simulink model "liner_two_wheel_model"  (R2018a)
settings: Solver=ode4  StartTime=0.0  StopTime=100  FixedStep=0.001  RelTol=1e-3
values from neighbouring files (symbols this model uses):
  CORNERING_POWER_OF_FRONT_TIRE = 200/(pi/180)    (= 11459.1559026)    [PARAMETERS.m]
  CORNERING_POWER_OF_REAR_TIRE = 200/(pi/180)    (= 11459.1559026)    [PARAMETERS.m]
  FRONT_SIDE_WHEELBASE = 0.8    [PARAMETERS.m]
  GEAR_RATIO = 14    [PARAMETERS.m]
  GRAVITATIONAL_ACCELERATION = 9.8    [PARAMETERS.m]
  HEIGHT_OF_GRAVITIONAL_CENTER = 0.3    [PARAMETERS.m]
  INITIAL_VELOCITY = TARGET_VELOCITY    (= 18)    [PARAMETERS.m]
  MAX_MOTOR_TORQUE = 21    [PARAMETERS.m]
  MAX_STEERING_ANGLE = 20/180*pi    (= 0.349065850399)    [PARAMETERS.m]
  REAR_SIDE_WHEELBASE = 0.7    [PARAMETERS.m]
  TIRE_RADIUS = 0.2286    [PARAMETERS.m]
  VEHICLE_MASS = 300    [PARAMETERS.m]
  VEHICLE_YAW_INERTIA = 120    [PARAMETERS.m]
  WHEELBASE = 1.5    [PARAMETERS.m]
libraries: simulink x1
settings Model: Creator=kntys  LastModifiedBy=kntys

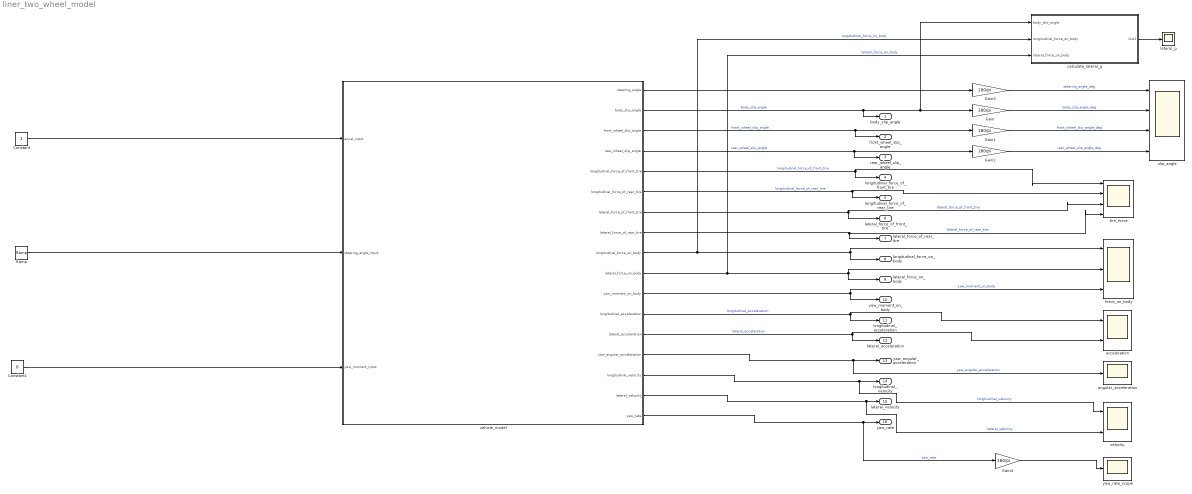
== system liner_two_wheel_model ==
  Constant : Constant
  Constant1 : Constant  Value=0
  Gain{,1..4} (5 alike) : Gain  Gain=180/pi
  Ramp : simulink/Sources/Ramp  slope=0.01  start=0  InitialOutput=0
  acceleration : Scope  NumInputPorts=2
  angular_acceleration : Scope
  calculate_lateral_g : Subsystem
  force_on_body : Scope  NumInputPorts=3
  lateral_g : Scope
  slip_angle : Scope  NumInputPorts=4
  tire_force : Scope  NumInputPorts=4
  vehicle_model : Subsystem
  velocity : Scope  NumInputPorts=2
  yaw_rate_scope : Scope
  body_slip_angle : Outport
  front_wheel_slip_angle : Outport  Port=2
  rear_wheel_slip_angle : Outport  Port=3
  longitudinal_force_of_front_tire : Outport  Port=4
  longitudinal_force_of_rear_tire : Outport  Port=5
  lateral_force_of_front_tire : Outport  Port=6
  lateral_force_of_rear_tire : Outport  Port=7
  longitudinal_force_on_body : Outport  Port=8
  lateral_force_on_body : Outport  Port=9
  yaw_moment_on_body : Outport  Port=10
  longitudinal_acceleration : Outport  Port=11
  lateral_acceleration : Outport  Port=12
  yaw_angular_acceleration : Outport  Port=13
  longitudinal_velocity : Outport  Port=14
  lateral_velocity : Outport  Port=15
  yaw_rate : Outport  Port=16
  wires:
  Ramp/1 -> vehicle_model/2(steering_angle_input)
  vehicle_model/16(lateral_velocity) -> velocity/2, lateral_velocity/1  "lateral_velocity"
  vehicle_model/15(longitudinal_velocity) -> velocity/1, longitudinal_velocity/1  "longitudinal_velocity"
  vehicle_model/17(yaw_rate) -> Gain4/1, yaw_rate/1  "yaw_rate"
  vehicle_model/2(body_slip_angle) -> body_slip_angle/1, calculate_lateral_g/1(body_slip_angle), Gain/1  "body_slip_angle"
  vehicle_model/3(front_wheel_slip_angle) -> front_wheel_slip_angle/1, Gain1/1  "front_wheel_slip_angle"
  vehicle_model/4(rear_wheel_slip_angle) -> rear_wheel_slip_angle/1, Gain2/1  "rear_wheel_slip_angle"
  vehicle_model/5(longitudinal_force_of_front_tire) -> longitudinal_force_of_front_tire/1, tire_force/1  "longitudinal_force_of_front_tire"
  vehicle_model/6(longitudinal_force_of_rear_tire) -> longitudinal_force_of_rear_tire/1, tire_force/2  "longitudinal_force_of_rear_tire"
  vehicle_model/7(lateral_force_of_front_tire) -> lateral_force_of_front_tire/1, tire_force/3  "lateral_force_of_front_tire"
  vehicle_model/8(lateral_force_of_rear_tire) -> lateral_force_of_rear_tire/1, tire_force/4  "lateral_force_of_rear_tire"
  vehicle_model/9(longitudinal_force_on_body) -> calculate_lateral_g/2(longitudinal_force_on_body), longitudinal_force_on_body/1, force_on_body/1  "longitudinal_force_on_body"
  vehicle_model/10(lateral_force_on_body) -> calculate_lateral_g/3(lateral_force_on_body), lateral_force_on_body/1, force_on_body/2  "lateral_force_on_body"
  vehicle_model/11(yaw_moment_on_body) -> yaw_moment_on_body/1, force_on_body/3  "yaw_moment_on_body"
  vehicle_model/12(longitudinal_acceleration) -> longitudinal_acceleration/1, acceleration/1  "longitudinal_acceleration"
  vehicle_model/13(lateral_acceleration) -> lateral_acceleration/1, acceleration/2  "lateral_acceleration"
  vehicle_model/14(yaw_angular_acceleration) -> angular_acceleration/1, yaw_angular_acceleration/1  "yaw_angular_acceleration"
  Constant1/1 -> vehicle_model/3(yaw_moment_input)
  Constant/1 -> vehicle_model/1(accel_input)
  Gain/1 -> slip_angle/2  "body_slip_angle_deg"
  Gain1/1 -> slip_angle/3  "front_wheel_slip_angle_deg"
  Gain2/1 -> slip_angle/4  "rear_wheel_slip_angle_deg"
  vehicle_model/1(steering_angle) -> Gain3/1
  Gain3/1 -> slip_angle/1  "steering_angle_deg"
  Gain4/1 -> yaw_rate_scope/1
  calculate_lateral_g/1(Out1) -> lateral_g/1

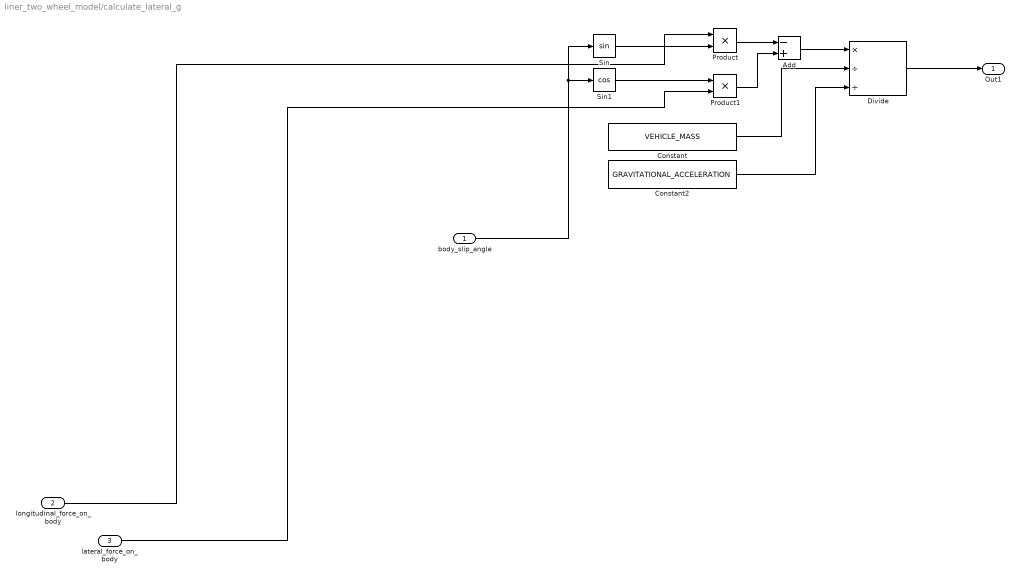
== system liner_two_wheel_model/calculate_lateral_g ==
  body_slip_angle : Inport
  longitudinal_force_on_body : Inport  Port=2
  lateral_force_on_body : Inport  Port=3
  Add : Sum  Inputs=-+
  Constant : Constant  Value=VEHICLE_MASS
  Constant2 : Constant  Value=GRAVITATIONAL_ACCELERATION
  Divide : Product  Inputs=*//
  Product : Product
  Product1 : Product
  Sin : Trigonometry
  Sin1 : Trigonometry  Operator=cos
  Out1 : Outport
  wires:
  body_slip_angle/1 -> Sin/1, Sin1/1
  Product/1 -> Add/1
  lateral_force_on_body/1 -> Product1/2
  Divide/1 -> Out1/1
  Add/1 -> Divide/1
  Constant2/1 -> Divide/3
  Sin1/1 -> Product1/1
  Constant/1 -> Divide/2
  Product1/1 -> Add/2
  Sin/1 -> Product/2
  longitudinal_force_on_body/1 -> Product/1

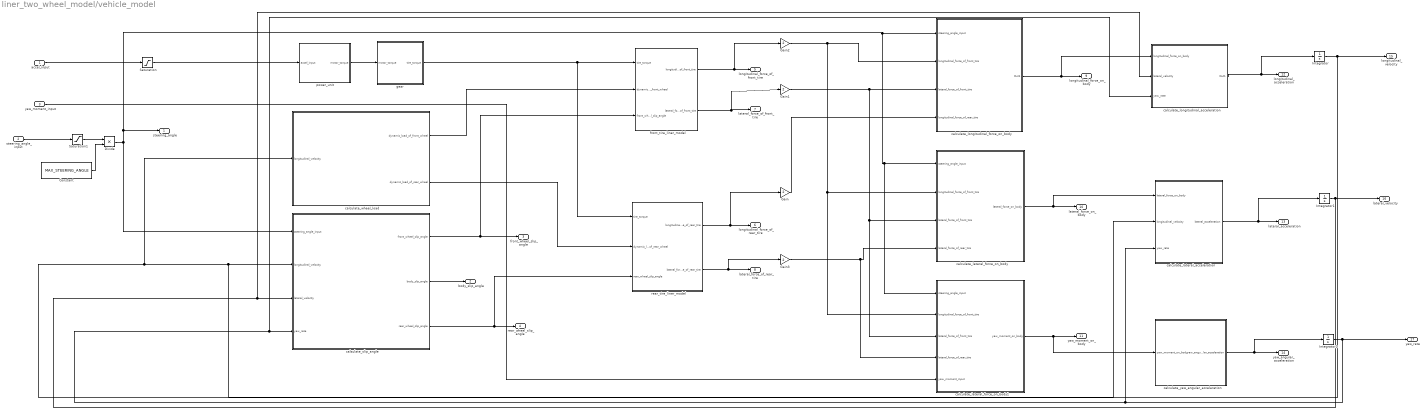
== system liner_two_wheel_model/vehicle_model ==
  accel_input : Inport
  steering_angle_input : Inport  Port=2
  yaw_moment_input : Inport  Port=3
  Constant : Constant  Value=MAX_STEERING_ANGLE
  Divide : Product  Inputs=**
  Gain{,1..3} (4 alike) : Gain  Gain=2
  Integrator : Integrator  InitialCondition=INITIAL_VELOCITY
  Integrator1 : Integrator
  Integrator2 : Integrator
  Saturation : Saturate  UpperLimit=1  LowerLimit=-1
  Saturation1 : Saturate  UpperLimit=1  LowerLimit=-1
  calculate_lateral_acceleration : Subsystem
  calculate_lateral_force_on_body : Subsystem
  calculate_lateral_force_on_body1 : Subsystem
  calculate_longitudinal_acceleration : Subsystem
  calculate_longitudinal_force_on_body : Subsystem
  calculate_wheel_load : Subsystem
  calculate_yaw_angular_accelaration : Subsystem
  calsulate_slip_angle : Subsystem
  front_tire_liner_model : Subsystem
  gear : Subsystem
  power_unit : Subsystem
  rear_tire_liner_model : Subsystem
  steering_angle : Outport
  body_slip_angle : Outport  Port=2
  front_wheel_slip_angle : Outport  Port=3
  rear_wheel_slip_angle : Outport  Port=4
  longitudinal_force_of_front_tire : Outport  Port=5
  longitudinal_force_of_rear_tire : Outport  Port=6
  lateral_force_of_front_tire : Outport  Port=7
  lateral_force_of_rear_tire : Outport  Port=8
  longitudinal_force_on_body : Outport  Port=9
  lateral_force_on_body : Outport  Port=10
  yaw_moment_on_body : Outport  Port=11
  longitudinal_acceleration : Outport  Port=12
  lateral_acceleration : Outport  Port=13
  yaw_angular_acceleration : Outport  Port=14
  longitudinal_velocity : Outport  Port=15
  lateral_velocity : Outport  Port=16
  yaw_rate : Outport  Port=17
  wires:
  accel_input/1 -> Saturation/1
  calculate_yaw_angular_accelaration/1(yaw_angular_acceleration) -> yaw_angular_acceleration/1, Integrator2/1
  Saturation/1 -> power_unit/1(accel_input)
  gear/1(tire_torque) -> rear_tire_liner_model/1(tire_torque), front_tire_liner_model/1(tire_torque)
  Gain/1 -> calculate_longitudinal_force_on_body/4(longitudinal_force_of_rear_tire)
  front_tire_liner_model/2(lateral_force_of_front_tire) -> lateral_force_of_front_tire/1, Gain1/1
  Gain2/1 -> calculate_lateral_force_on_body1/2(longitudinal_force_of_front_tire), calculate_lateral_force_on_body/2(longitudinal_force_of_front_tire), calculate_longitudinal_force_on_body/2(longitudinal_force_of_front_tire)
  calsulate_slip_angle/3(rear_wheel_slip_angle) -> rear_wheel_slip_angle/1, rear_tire_liner_model/3(rear_wheel_slip_angle)
  calculate_lateral_acceleration/1(lateral_acceleration) -> lateral_acceleration/1, Integrator1/1
  front_tire_liner_model/1(longitudinal_force_of_front_tire) -> longitudinal_force_of_front_tire/1, Gain2/1
  calsulate_slip_angle/1(front_wheel_slip_angle) -> front_wheel_slip_angle/1, front_tire_liner_model/3(front_wheel_slip_angle)
  Divide/1 -> calsulate_slip_angle/1(steering_angle_input), steering_angle/1, calculate_lateral_force_on_body1/1(steering_angle_input), calculate_lateral_force_on_body/1(steering_angle_input), calculate_longitudinal_force_on_body/1(steering_angle_input)
  calculate_longitudinal_acceleration/1(Out1) -> longitudinal_acceleration/1, Integrator/1
  calculate_wheel_load/2(dynamic_load_of_rear_wheel) -> rear_tire_liner_model/2(dynamic_load_of_rear_wheel)
  Integrator2/1 -> calculate_longitudinal_acceleration/3(yaw_rate), calsulate_slip_angle/4(yaw_rate), calculate_lateral_acceleration/3(yaw_rate), yaw_rate/1
  calculate_wheel_load/1(dynamic_load_of_front_wheel) -> front_tire_liner_model/2(dynamic_load_of_front_wheel)
  calsulate_slip_angle/2(body_slip_angle) -> body_slip_angle/1
  rear_tire_liner_model/2(lateral_force_of_rear_tire) -> lateral_force_of_rear_tire/1, Gain3/1
  Gain3/1 -> calculate_lateral_force_on_body1/4(lateral_force_of_rear_tire), calculate_lateral_force_on_body/4(lateral_force_of_rear_tire)
  rear_tire_liner_model/1(longitudinal_force_of_rear_tire) -> longitudinal_force_of_rear_tire/1, Gain/1
  calculate_lateral_force_on_body1/1(yaw_moment_on_body) -> yaw_moment_on_body/1, calculate_yaw_angular_accelaration/1(yaw_moment_on_body)
  Gain1/1 -> calculate_lateral_force_on_body1/3(lateral_force_of_front_tire), calculate_lateral_force_on_body/3(lateral_force_of_front_tire), calculate_longitudinal_force_on_body/3(lateral_force_of_front_tire)
  Integrator/1 -> longitudinal_velocity/1, calculate_wheel_load/1(longitudinal_velocity), calculate_lateral_acceleration/2(longitudinal_velocity), calsulate_slip_angle/2(longitudinal_velocity)
  calculate_lateral_force_on_body/1(lateral_force_on_body) -> lateral_force_on_body/1, calculate_lateral_acceleration/1(lateral_force_on_body)
  Integrator1/1 -> lateral_velocity/1, calculate_longitudinal_acceleration/2(lateral_velocity), calsulate_slip_angle/3(lateral_velocity)
  calculate_longitudinal_force_on_body/1(Out1) -> longitudinal_force_on_body/1, calculate_longitudinal_acceleration/1(longitudinal_force_on_body)
  yaw_moment_input/1 -> calculate_lateral_force_on_body1/5(yaw_moment_input)
  power_unit/1(motor_torque) -> gear/1(motor_torque)
  steering_angle_input/1 -> Saturation1/1
  Constant/1 -> Divide/2
  Saturation1/1 -> Divide/1

== system liner_two_wheel_model/vehicle_model/calculate_lateral_acceleration ==
  lateral_force_on_body : Inport
  longitudinal_velocity : Inport  Port=2
  yaw_rate : Inport  Port=3
  Add1 : Sum  Inputs=+-
  Constant1 : Constant  Value=VEHICLE_MASS
  Divide : Product  Inputs=*/
  Divide3 : Product  Inputs=**
  lateral_acceleration : Outport
  wires:
  longitudinal_velocity/1 -> Divide3/1
  Divide/1 -> Add1/1
  lateral_force_on_body/1 -> Divide/1
  Constant1/1 -> Divide/2
  yaw_rate/1 -> Divide3/2
  Add1/1 -> lateral_acceleration/1
  Divide3/1 -> Add1/2

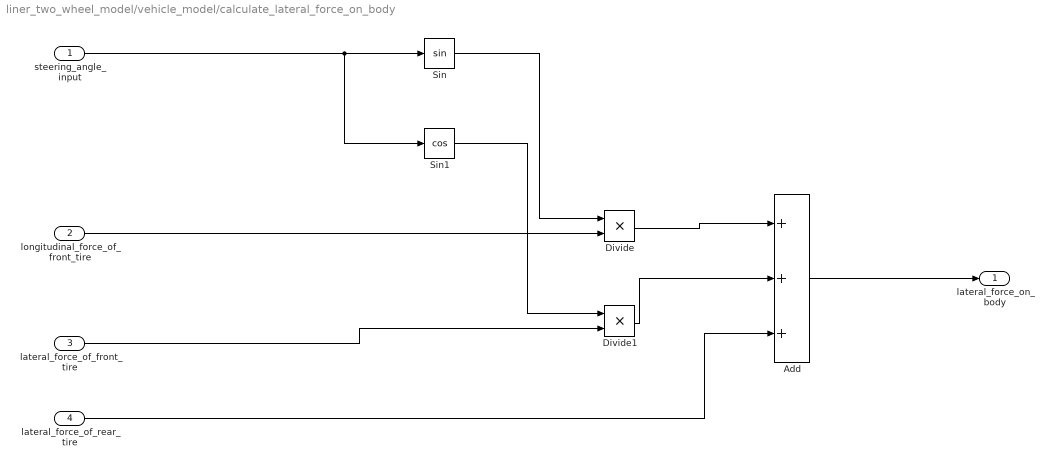
== system liner_two_wheel_model/vehicle_model/calculate_lateral_force_on_body ==
  steering_angle_input : Inport
  longitudinal_force_of_front_tire : Inport  Port=2
  lateral_force_of_front_tire : Inport  Port=3
  lateral_force_of_rear_tire : Inport  Port=4
  Add : Sum  Inputs=+++
  Divide : Product  Inputs=**
  Divide1 : Product  Inputs=**
  Sin : Trigonometry
  Sin1 : Trigonometry  Operator=cos
  lateral_force_on_body : Outport
  wires:
  longitudinal_force_of_front_tire/1 -> Divide/2
  steering_angle_input/1 -> Sin/1, Sin1/1
  Divide/1 -> Add/1
  Add/1 -> lateral_force_on_body/1
  Divide1/1 -> Add/2
  Sin1/1 -> Divide1/1
  Sin/1 -> Divide/1
  lateral_force_of_front_tire/1 -> Divide1/2
  lateral_force_of_rear_tire/1 -> Add/3

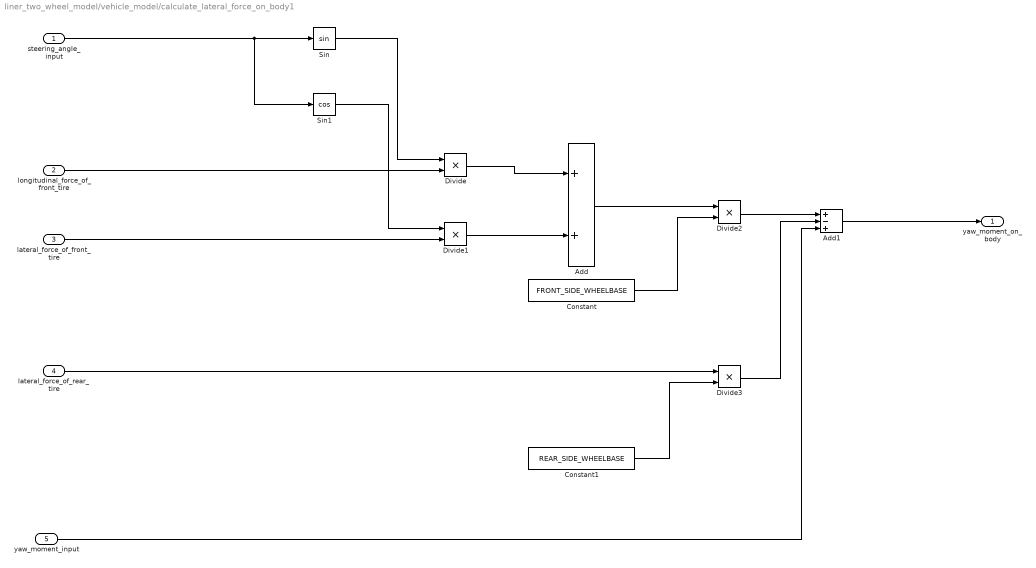
== system liner_two_wheel_model/vehicle_model/calculate_lateral_force_on_body1 ==
  steering_angle_input : Inport
  longitudinal_force_of_front_tire : Inport  Port=2
  lateral_force_of_front_tire : Inport  Port=3
  lateral_force_of_rear_tire : Inport  Port=4
  yaw_moment_input : Inport  Port=5
  Add : Sum
  Add1 : Sum  Inputs=+-+
  Constant : Constant  Value=FRONT_SIDE_WHEELBASE
  Constant1 : Constant  Value=REAR_SIDE_WHEELBASE
  Divide{,1..3} (4 alike) : Product  Inputs=**
  Sin : Trigonometry
  Sin1 : Trigonometry  Operator=cos
  yaw_moment_on_body : Outport
  wires:
  longitudinal_force_of_front_tire/1 -> Divide/2
  steering_angle_input/1 -> Sin/1, Sin1/1
  Divide/1 -> Add/1
  Add/1 -> Divide2/1
  Divide1/1 -> Add/2
  Sin1/1 -> Divide1/1
  Sin/1 -> Divide/1
  lateral_force_of_front_tire/1 -> Divide1/2
  lateral_force_of_rear_tire/1 -> Divide3/1
  Constant/1 -> Divide2/2
  Divide2/1 -> Add1/1
  Divide3/1 -> Add1/2
  Constant1/1 -> Divide3/2
  yaw_moment_input/1 -> Add1/3
  Add1/1 -> yaw_moment_on_body/1

== system liner_two_wheel_model/vehicle_model/calculate_longitudinal_acceleration ==
  longitudinal_force_on_body : Inport
  lateral_velocity : Inport  Port=2
  yaw_rate : Inport  Port=3
  Add : Sum
  Constant : Constant  Value=VEHICLE_MASS
  Divide1 : Product  Inputs=*/
  Divide2 : Product  Inputs=**
  Out1 : Outport
  wires:
  Divide1/1 -> Add/1
  longitudinal_force_on_body/1 -> Divide1/1
  lateral_velocity/1 -> Divide2/1
  Divide2/1 -> Add/2
  yaw_rate/1 -> Divide2/2
  Constant/1 -> Divide1/2
  Add/1 -> Out1/1

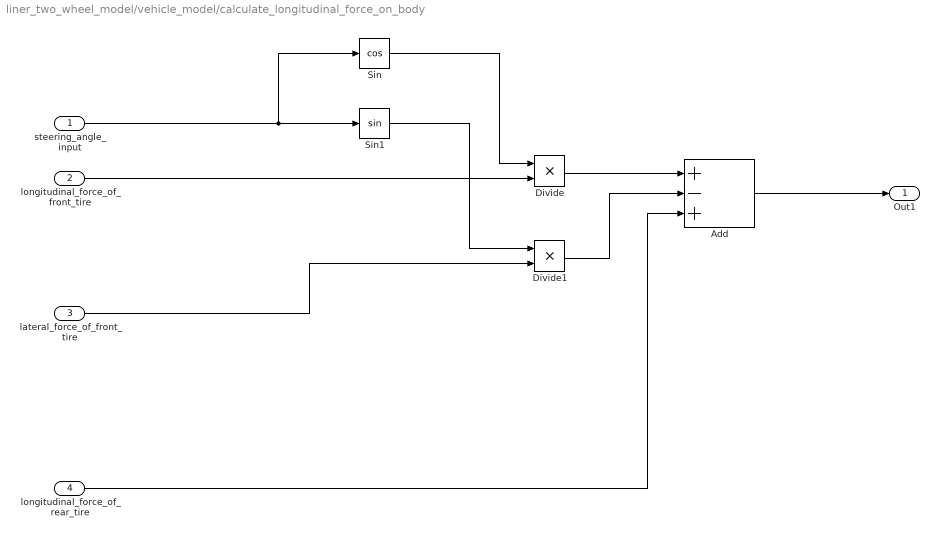
== system liner_two_wheel_model/vehicle_model/calculate_longitudinal_force_on_body ==
  steering_angle_input : Inport
  longitudinal_force_of_front_tire : Inport  Port=2
  lateral_force_of_front_tire : Inport  Port=3
  longitudinal_force_of_rear_tire : Inport  Port=4
  Add : Sum  Inputs=+-+
  Divide : Product  Inputs=**
  Divide1 : Product  Inputs=**
  Sin : Trigonometry  Operator=cos
  Sin1 : Trigonometry
  Out1 : Outport
  wires:
  steering_angle_input/1 -> Sin/1, Sin1/1
  Add/1 -> Out1/1
  Divide1/1 -> Add/2
  Sin/1 -> Divide/1
  longitudinal_force_of_rear_tire/1 -> Add/3
  Divide/1 -> Add/1
  lateral_force_of_front_tire/1 -> Divide1/2
  Sin1/1 -> Divide1/1
  longitudinal_force_of_front_tire/1 -> Divide/2

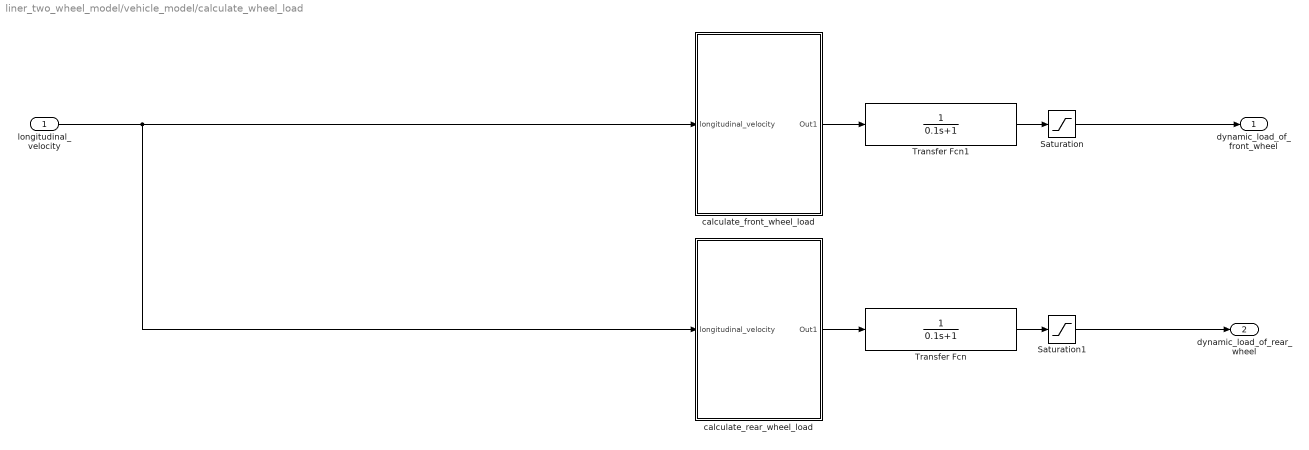
== system liner_two_wheel_model/vehicle_model/calculate_wheel_load ==
  longitudinal_velocity : Inport
  Saturation : Saturate  UpperLimit=inf  LowerLimit=0
  Saturation1 : Saturate  UpperLimit=inf  LowerLimit=0
  Transfer Fcn : TransferFcn  Denominator=[0.1 1]
  Transfer Fcn1 : TransferFcn  Denominator=[0.1 1]
  calculate_front_wheel_load : Subsystem
  calculate_rear_wheel_load : Subsystem
  dynamic_load_of_front_wheel : Outport
  dynamic_load_of_rear_wheel : Outport  Port=2
  wires:
  longitudinal_velocity/1 -> calculate_rear_wheel_load/1(longitudinal_velocity), calculate_front_wheel_load/1(longitudinal_velocity)
  calculate_rear_wheel_load/1(Out1) -> Transfer Fcn/1
  calculate_front_wheel_load/1(Out1) -> Transfer Fcn1/1
  Saturation/1 -> dynamic_load_of_front_wheel/1
  Saturation1/1 -> dynamic_load_of_rear_wheel/1
  Transfer Fcn1/1 -> Saturation/1
  Transfer Fcn/1 -> Saturation1/1

== system liner_two_wheel_model/vehicle_model/calculate_yaw_angular_accelaration ==
  yaw_moment_on_body : Inport
  Constant2 : Constant  Value=VEHICLE_YAW_INERTIA
  Divide4 : Product  Inputs=*/
  yaw_angular_acceleration : Outport
  wires:
  Constant2/1 -> Divide4/2
  Divide4/1 -> yaw_angular_acceleration/1
  yaw_moment_on_body/1 -> Divide4/1

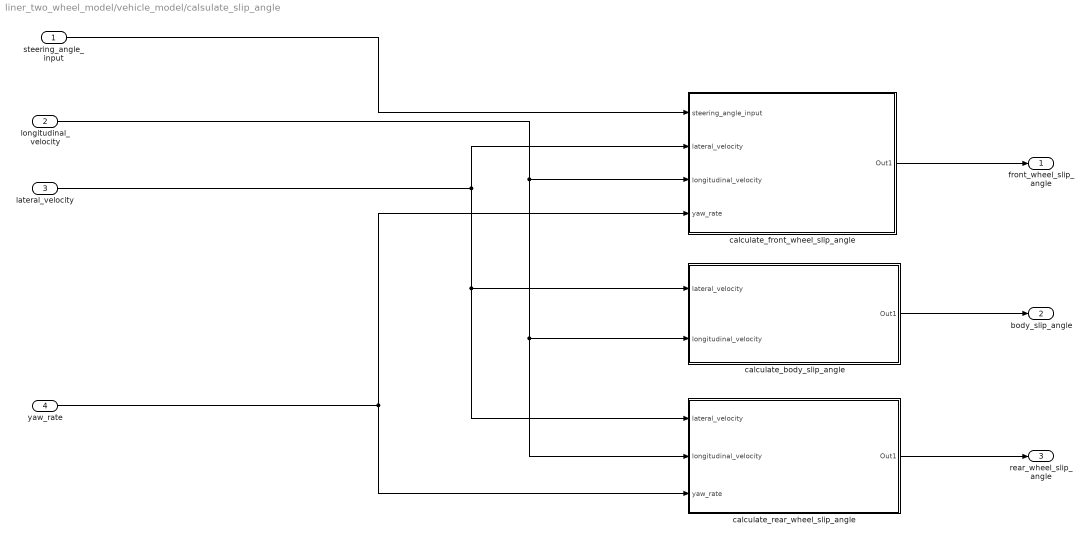
== system liner_two_wheel_model/vehicle_model/calsulate_slip_angle ==
  steering_angle_input : Inport
  longitudinal_velocity : Inport  Port=2
  lateral_velocity : Inport  Port=3
  yaw_rate : Inport  Port=4
  calculate_body_slip_angle : Subsystem
  "calculate_front_wheel_slip_angle " : Subsystem
  "calculate_rear_wheel_slip_angle " : Subsystem
  front_wheel_slip_angle : Outport
  body_slip_angle : Outport  Port=2
  rear_wheel_slip_angle : Outport  Port=3
  wires:
  lateral_velocity/1 -> "calculate_front_wheel_slip_angle "/2(lateral_velocity), calculate_body_slip_angle/1(lateral_velocity), "calculate_rear_wheel_slip_angle "/1(lateral_velocity)
  longitudinal_velocity/1 -> calculate_body_slip_angle/2(longitudinal_velocity), "calculate_rear_wheel_slip_angle "/2(longitudinal_velocity), "calculate_front_wheel_slip_angle "/3(longitudinal_velocity)
  "calculate_front_wheel_slip_angle "/1(Out1) -> front_wheel_slip_angle/1
  yaw_rate/1 -> "calculate_front_wheel_slip_angle "/4(yaw_rate), "calculate_rear_wheel_slip_angle "/3(yaw_rate)
  "calculate_rear_wheel_slip_angle "/1(Out1) -> rear_wheel_slip_angle/1
  calculate_body_slip_angle/1(Out1) -> body_slip_angle/1
  steering_angle_input/1 -> "calculate_front_wheel_slip_angle "/1(steering_angle_input)

== system liner_two_wheel_model/vehicle_model/front_tire_liner_model ==
  tire_torque : Inport
  dynamic_load_of_front_wheel : Inport  Port=2
  front_wheel_slip_angle : Inport  Port=3
  calculate_lateral_force_of_front_tire : Subsystem
  calculate_longitudinal_force_of_front_tire : Subsystem
  longitudinal_force_of_front_tire : Outport
  lateral_force_of_front_tire : Outport  Port=2
  wires:
  dynamic_load_of_front_wheel/1 -> calculate_lateral_force_of_front_tire/1(dynamic_load_of_front_wheel), calculate_longitudinal_force_of_front_tire/2(dynamic_load_of_front_wheel)
  tire_torque/1 -> calculate_longitudinal_force_of_front_tire/1(tire_torque)
  calculate_longitudinal_force_of_front_tire/1(longitudinal_force_of_front_tire) -> longitudinal_force_of_front_tire/1
  front_wheel_slip_angle/1 -> calculate_lateral_force_of_front_tire/2(front_wheel_slip_angle)
  calculate_lateral_force_of_front_tire/1(lateral_force_of_front_tire) -> lateral_force_of_front_tire/1

== system liner_two_wheel_model/vehicle_model/gear ==
  motor_torque : Inport
  Constant1 : Constant  Value=GEAR_RATIO
  Divide1 : Product  Inputs=**
  tire_torque : Outport
  wires:
  Constant1/1 -> Divide1/1
  motor_torque/1 -> Divide1/2
  Divide1/1 -> tire_torque/1

== system liner_two_wheel_model/vehicle_model/power_unit ==
  accel_input : Inport
  Constant : Constant  Value=MAX_MOTOR_TORQUE
  Divide : Product  Inputs=**
  motor_torque : Outport
  wires:
  Divide/1 -> motor_torque/1
  Constant/1 -> Divide/1
  accel_input/1 -> Divide/2

== system liner_two_wheel_model/vehicle_model/rear_tire_liner_model ==
  tire_torque : Inport
  dynamic_load_of_rear_wheel : Inport  Port=2
  rear_wheel_slip_angle : Inport  Port=3
  calculate_lateral_force_of_rear_tire : Subsystem
  calculate_longitudinal_force_of_rear_tire : Subsystem
  longitudinal_force_of_rear_tire : Outport
  lateral_force_of_rear_tire : Outport  Port=2
  wires:
  dynamic_load_of_rear_wheel/1 -> calculate_lateral_force_of_rear_tire/2(dynamic_load_of_rear_wheel), calculate_longitudinal_force_of_rear_tire/2(dynamic_load_of_rear_wheel)
  rear_wheel_slip_angle/1 -> calculate_lateral_force_of_rear_tire/1(rear_wheel_slip_angle)
  calculate_longitudinal_force_of_rear_tire/1(longitudinal_force_of_rear_tire) -> longitudinal_force_of_rear_tire/1
  calculate_lateral_force_of_rear_tire/1(lateral_force_of_rear_tire) -> lateral_force_of_rear_tire/1
  tire_torque/1 -> calculate_longitudinal_force_of_rear_tire/1(tire_torque)

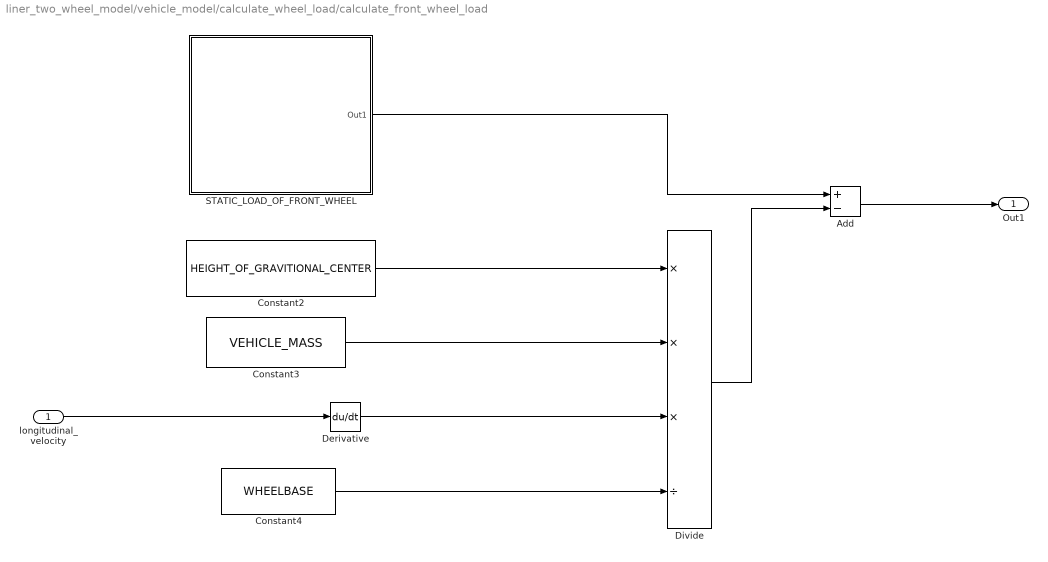
== system liner_two_wheel_model/vehicle_model/calculate_wheel_load/calculate_front_wheel_load ==
  longitudinal_velocity : Inport
  Add : Sum  Inputs=+-
  Constant2 : Constant  Value=HEIGHT_OF_GRAVITIONAL_CENTER
  Constant3 : Constant  Value=VEHICLE_MASS
  Constant4 : Constant  Value=WHEELBASE
  Derivative : Derivative
  Divide : Product  Inputs=***/
  STATIC_LOAD_OF_FRONT_WHEEL : Subsystem
  Out1 : Outport
  wires:
  longitudinal_velocity/1 -> Derivative/1
  Constant3/1 -> Divide/2
  Constant4/1 -> Divide/4
  STATIC_LOAD_OF_FRONT_WHEEL/1(Out1) -> Add/1
  Divide/1 -> Add/2
  Constant2/1 -> Divide/1
  Add/1 -> Out1/1
  Derivative/1 -> Divide/3

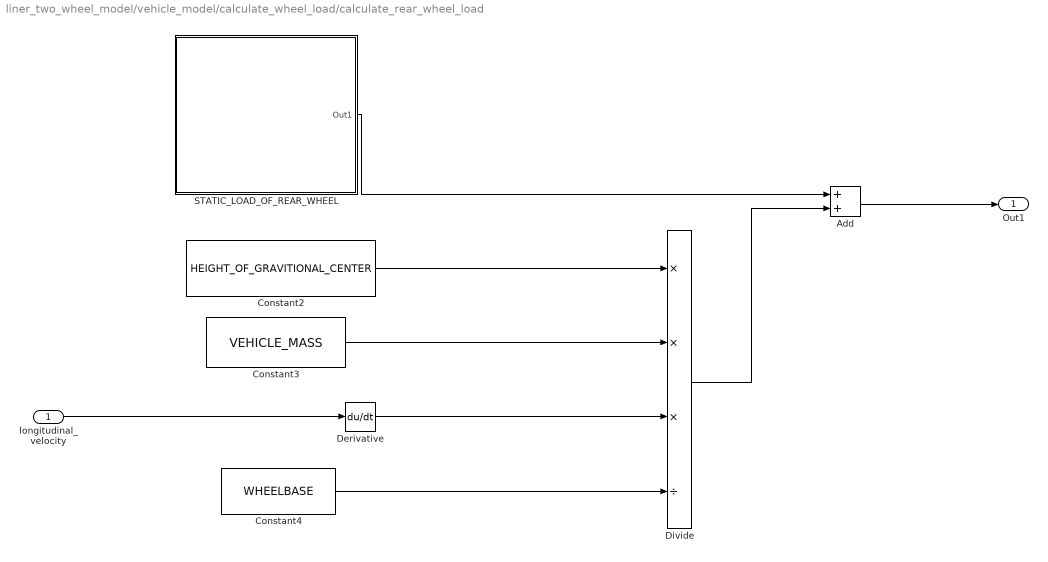
== system liner_two_wheel_model/vehicle_model/calculate_wheel_load/calculate_rear_wheel_load ==
  longitudinal_velocity : Inport
  Add : Sum
  Constant2 : Constant  Value=HEIGHT_OF_GRAVITIONAL_CENTER
  Constant3 : Constant  Value=VEHICLE_MASS
  Constant4 : Constant  Value=WHEELBASE
  Derivative : Derivative
  Divide : Product  Inputs=***/
  STATIC_LOAD_OF_REAR_WHEEL : Subsystem
  Out1 : Outport
  wires:
  longitudinal_velocity/1 -> Derivative/1
  Constant3/1 -> Divide/2
  Constant4/1 -> Divide/4
  STATIC_LOAD_OF_REAR_WHEEL/1(Out1) -> Add/1
  Divide/1 -> Add/2
  Constant2/1 -> Divide/1
  Add/1 -> Out1/1
  Derivative/1 -> Divide/3

== system liner_two_wheel_model/vehicle_model/calsulate_slip_angle/calculate_body_slip_angle ==
  lateral_velocity : Inport
  longitudinal_velocity : Inport  Port=2
  Divide : Product  Inputs=*/
  arctan : Trigonometry  Operator=atan
  Out1 : Outport
  wires:
  longitudinal_velocity/1 -> Divide/2
  Divide/1 -> arctan/1
  lateral_velocity/1 -> Divide/1
  arctan/1 -> Out1/1

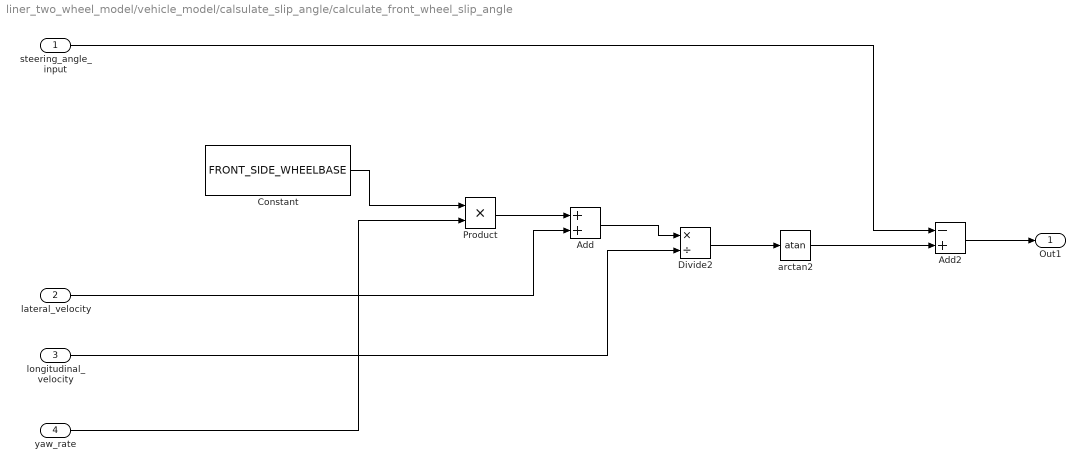
== system liner_two_wheel_model/vehicle_model/calsulate_slip_angle/calculate_front_wheel_slip_angle  ==
  steering_angle_input : Inport
  lateral_velocity : Inport  Port=2
  longitudinal_velocity : Inport  Port=3
  yaw_rate : Inport  Port=4
  Add : Sum
  Add2 : Sum  Inputs=-+
  Constant : Constant  Value=FRONT_SIDE_WHEELBASE
  Divide2 : Product  Inputs=*/
  Product : Product
  arctan2 : Trigonometry  Operator=atan
  Out1 : Outport
  wires:
  Product/1 -> Add/1
  longitudinal_velocity/1 -> Divide2/2
  Add/1 -> Divide2/1
  arctan2/1 -> Add2/2
  Divide2/1 -> arctan2/1
  lateral_velocity/1 -> Add/2
  yaw_rate/1 -> Product/2
  Constant/1 -> Product/1
  steering_angle_input/1 -> Add2/1
  Add2/1 -> Out1/1

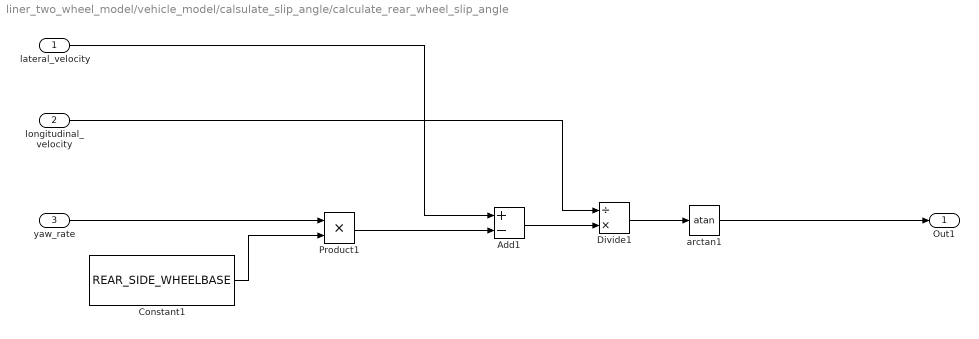
== system liner_two_wheel_model/vehicle_model/calsulate_slip_angle/calculate_rear_wheel_slip_angle  ==
  lateral_velocity : Inport
  longitudinal_velocity : Inport  Port=2
  yaw_rate : Inport  Port=3
  Add1 : Sum  Inputs=+-
  Constant1 : Constant  Value=REAR_SIDE_WHEELBASE
  Divide1 : Product  Inputs=/*
  Product1 : Product
  arctan1 : Trigonometry  Operator=atan
  Out1 : Outport
  wires:
  Divide1/1 -> arctan1/1
  Product1/1 -> Add1/2
  longitudinal_velocity/1 -> Divide1/1
  Add1/1 -> Divide1/2
  Constant1/1 -> Product1/2
  yaw_rate/1 -> Product1/1
  arctan1/1 -> Out1/1
  lateral_velocity/1 -> Add1/1

== system liner_two_wheel_model/vehicle_model/front_tire_liner_model/calculate_lateral_force_of_front_tire ==
  dynamic_load_of_front_wheel : Inport
  front_wheel_slip_angle : Inport  Port=2
  Constant : Constant  Value=CORNERING_POWER_OF_FRONT_TIRE
  Divide : Product  Inputs=***/
  Gain : Gain  Gain=-1
  STATIC_LOAD_OF_FRONT_WHEEL : Subsystem
  Transfer Fcn : TransferFcn  Denominator=[0.01 1]
  lateral_force_of_front_tire : Outport
  wires:
  STATIC_LOAD_OF_FRONT_WHEEL/1(Out1) -> Divide/4
  front_wheel_slip_angle/1 -> Transfer Fcn/1
  Gain/1 -> Divide/1
  Constant/1 -> Gain/1
  Divide/1 -> lateral_force_of_front_tire/1
  dynamic_load_of_front_wheel/1 -> Divide/3
  Transfer Fcn/1 -> Divide/2

== system liner_two_wheel_model/vehicle_model/front_tire_liner_model/calculate_longitudinal_force_of_front_tire ==
  tire_torque : Inport
  dynamic_load_of_front_wheel : Inport  Port=2
  Constant : Constant  Value=TIRE_RADIUS
  Divide : Product  Inputs=*/
  Divide1 : Product  Inputs=**/
  STATIC_LOAD_OF_FRONT_WHEEL : Subsystem
  longitudinal_force_of_front_tire : Outport
  wires:
  Divide1/1 -> longitudinal_force_of_front_tire/1
  STATIC_LOAD_OF_FRONT_WHEEL/1(Out1) -> Divide1/3
  Divide/1 -> Divide1/1
  Constant/1 -> Divide/2
  dynamic_load_of_front_wheel/1 -> Divide1/2
  tire_torque/1 -> Divide/1

== system liner_two_wheel_model/vehicle_model/rear_tire_liner_model/calculate_lateral_force_of_rear_tire ==
  rear_wheel_slip_angle : Inport
  dynamic_load_of_rear_wheel : Inport  Port=2
  Constant : Constant  Value=CORNERING_POWER_OF_REAR_TIRE
  Divide : Product  Inputs=***/
  Gain : Gain  Gain=-1
  STATIC_LOAD_OF_REAR_WHEEL : Subsystem
  Transfer Fcn : TransferFcn  Denominator=[0.01 1]
  lateral_force_of_rear_tire : Outport
  wires:
  STATIC_LOAD_OF_REAR_WHEEL/1(Out1) -> Divide/4
  Gain/1 -> Divide/1
  rear_wheel_slip_angle/1 -> Transfer Fcn/1
  Constant/1 -> Gain/1
  Divide/1 -> lateral_force_of_rear_tire/1
  dynamic_load_of_rear_wheel/1 -> Divide/3
  Transfer Fcn/1 -> Divide/2

== system liner_two_wheel_model/vehicle_model/rear_tire_liner_model/calculate_longitudinal_force_of_rear_tire ==
  tire_torque : Inport
  dynamic_load_of_rear_wheel : Inport  Port=2
  Constant : Constant  Value=TIRE_RADIUS
  Divide : Product  Inputs=*/
  Divide1 : Product  Inputs=**/
  STATIC_LOAD_OF_REAR_WHEEL : Subsystem
  longitudinal_force_of_rear_tire : Outport
  wires:
  STATIC_LOAD_OF_REAR_WHEEL/1(Out1) -> Divide1/3
  Constant/1 -> Divide/2
  Divide1/1 -> longitudinal_force_of_rear_tire/1
  Divide/1 -> Divide1/1
  dynamic_load_of_rear_wheel/1 -> Divide1/2
  tire_torque/1 -> Divide/1

== system liner_two_wheel_model/vehicle_model/calculate_wheel_load/calculate_front_wheel_load/STATIC_LOAD_OF_FRONT_WHEEL ==
  Constant1 : Constant  Value=REAR_SIDE_WHEELBASE
  Constant2 : Constant  Value=GRAVITATIONAL_ACCELERATION
  Constant3 : Constant  Value=VEHICLE_MASS
  Constant4 : Constant  Value=WHEELBASE
  Divide2 : Product  Inputs=***/
  Out1 : Outport
  wires:
  Divide2/1 -> Out1/1
  Constant4/1 -> Divide2/4
  Constant3/1 -> Divide2/1
  Constant1/1 -> Divide2/2
  Constant2/1 -> Divide2/3

== system liner_two_wheel_model/vehicle_model/calculate_wheel_load/calculate_rear_wheel_load/STATIC_LOAD_OF_REAR_WHEEL ==
  Constant1 : Constant  Value=FRONT_SIDE_WHEELBASE
  Constant2 : Constant  Value=GRAVITATIONAL_ACCELERATION
  Constant3 : Constant  Value=VEHICLE_MASS
  Constant4 : Constant  Value=WHEELBASE
  Divide2 : Product  Inputs=***/
  Out1 : Outport
  wires:
  Divide2/1 -> Out1/1
  Constant4/1 -> Divide2/4
  Constant3/1 -> Divide2/1
  Constant1/1 -> Divide2/2
  Constant2/1 -> Divide2/3

== system liner_two_wheel_model/vehicle_model/front_tire_liner_model/calculate_lateral_force_of_front_tire/STATIC_LOAD_OF_FRONT_WHEEL ==
  Constant1 : Constant  Value=REAR_SIDE_WHEELBASE
  Constant2 : Constant  Value=GRAVITATIONAL_ACCELERATION
  Constant3 : Constant  Value=VEHICLE_MASS
  Constant4 : Constant  Value=WHEELBASE
  Divide2 : Product  Inputs=***/
  Out1 : Outport
  wires:
  Divide2/1 -> Out1/1
  Constant4/1 -> Divide2/4
  Constant3/1 -> Divide2/1
  Constant1/1 -> Divide2/2
  Constant2/1 -> Divide2/3

== system liner_two_wheel_model/vehicle_model/front_tire_liner_model/calculate_longitudinal_force_of_front_tire/STATIC_LOAD_OF_FRONT_WHEEL ==
  Constant1 : Constant  Value=REAR_SIDE_WHEELBASE
  Constant2 : Constant  Value=GRAVITATIONAL_ACCELERATION
  Constant3 : Constant  Value=VEHICLE_MASS
  Constant4 : Constant  Value=WHEELBASE
  Divide2 : Product  Inputs=***/
  Out1 : Outport
  wires:
  Divide2/1 -> Out1/1
  Constant4/1 -> Divide2/4
  Constant3/1 -> Divide2/1
  Constant1/1 -> Divide2/2
  Constant2/1 -> Divide2/3

== system liner_two_wheel_model/vehicle_model/rear_tire_liner_model/calculate_lateral_force_of_rear_tire/STATIC_LOAD_OF_REAR_WHEEL ==
  Constant1 : Constant  Value=FRONT_SIDE_WHEELBASE
  Constant2 : Constant  Value=GRAVITATIONAL_ACCELERATION
  Constant3 : Constant  Value=VEHICLE_MASS
  Constant4 : Constant  Value=WHEELBASE
  Divide2 : Product  Inputs=***/
  Out1 : Outport
  wires:
  Divide2/1 -> Out1/1
  Constant4/1 -> Divide2/4
  Constant3/1 -> Divide2/1
  Constant1/1 -> Divide2/2
  Constant2/1 -> Divide2/3

== system liner_two_wheel_model/vehicle_model/rear_tire_liner_model/calculate_longitudinal_force_of_rear_tire/STATIC_LOAD_OF_REAR_WHEEL ==
  Constant1 : Constant  Value=FRONT_SIDE_WHEELBASE
  Constant2 : Constant  Value=GRAVITATIONAL_ACCELERATION
  Constant3 : Constant  Value=VEHICLE_MASS
  Constant4 : Constant  Value=WHEELBASE
  Divide2 : Product  Inputs=***/
  Out1 : Outport
  wires:
  Divide2/1 -> Out1/1
  Constant4/1 -> Divide2/4
  Constant3/1 -> Divide2/1
  Constant1/1 -> Divide2/2
  Constant2/1 -> Divide2/3
